simulink model "P2"  (R2019a)
settings: Solver=VariableStepAuto  StartTime=0.0  StopTime=50.0  RelTol=1e-3
libraries: simulink x8
settings Model: Creator=ADMIN  LastModifiedBy=ADMIN

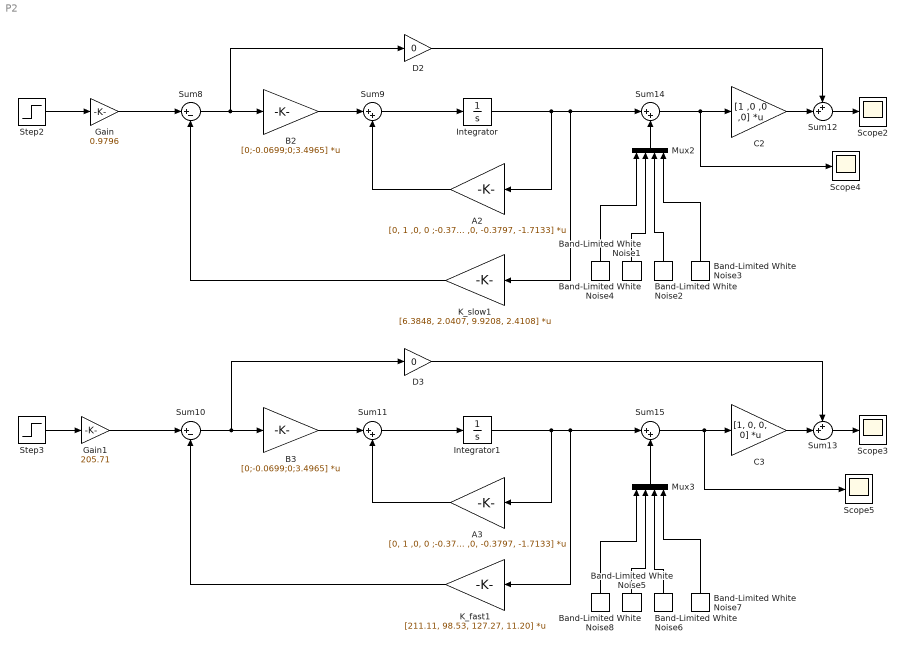
== system P2 ==
  A2 : Gain  Gain=[0, 1 ,0, 0 ;-0.378 ,0 ,7.0147 ,0.0343;0, 0, 0, 1; 18.9001 ,0, -0.3797, -1.7133]  Multiplication=Matrix(K*u) (u vector)
  A3 : Gain  Gain=[0, 1 ,0, 0 ;-0.378 ,0 ,7.0147 ,0.0343;0, 0, 0, 1; 18.9001 ,0, -0.3797, -1.7133]  Multiplication=Matrix(K*u) (u vector)
  B2 : Gain  Gain=[0;-0.0699;0;3.4965]  Multiplication=Matrix(K*u) (u vector)
  B3 : Gain  Gain=[0;-0.0699;0;3.4965]  Multiplication=Matrix(K*u) (u vector)
  Band-Limited White Noise1 : simulink/Sources/Band-Limited White Noise  Cov=[1e-5]  Ts=10  seed=2525
  Band-Limited White Noise2 : simulink/Sources/Band-Limited White Noise  Cov=[1e-5]  Ts=10  seed=[23341]
  Band-Limited White Noise3 : simulink/Sources/Band-Limited White Noise  Cov=[1e-5]  Ts=10  seed=[2342]
  Band-Limited White Noise4 : simulink/Sources/Band-Limited White Noise  Cov=[1e-5]  Ts=10  seed=[3]
  Band-Limited White Noise5 : simulink/Sources/Band-Limited White Noise  Cov=[1e-5]  Ts=10  seed=2525
  Band-Limited White Noise6 : simulink/Sources/Band-Limited White Noise  Cov=[1e-5]  Ts=10  seed=[23341]
  Band-Limited White Noise7 : simulink/Sources/Band-Limited White Noise  Cov=[1e-5]  Ts=10  seed=[2342]
  Band-Limited White Noise8 : simulink/Sources/Band-Limited White Noise  Cov=[1e-5]  Ts=10  seed=[3]
  C2 : Gain  Gain=[1 ,0 ,0 ,0]  Multiplication=Matrix(K*u) (u vector)
  C3 : Gain  Gain=[1, 0, 0, 0]  Multiplication=Matrix(K*u) (u vector)
  D2 : Gain  Gain=0
  D3 : Gain  Gain=0
  Gain : Gain  Gain=0.9796
  Gain1 : Gain  Gain=205.71
  Integrator : Integrator
  Integrator1 : Integrator
  K_fast1 : Gain  Gain=[211.11, 98.53, 127.27, 11.20]  Multiplication=Matrix(K*u) (u vector)
  K_slow1 : Gain  Gain=[6.3848, 2.0407, 9.9208, 2.4108]  Multiplication=Matrix(K*u) (u vector)
  Mux2 : Mux
  Mux3 : Mux
  Scope{2..5} (4 alike) : Scope
  Step2 : Step  Time=0  After=0.1  SampleTime=0
  Step3 : Step  Time=0  After=0.1  SampleTime=0
  Sum10 : Sum  Inputs=|+-
  Sum{9,11,14..15} (4 alike) : Sum  Inputs=|++
  Sum12 : Sum  Inputs=++|
  Sum13 : Sum  Inputs=++|
  Sum8 : Sum  Inputs=|+-
  wires:
  Sum8/1 -> B2/1, D2/1
  Sum11/1 -> Integrator1/1
  Gain/1 -> Sum8/1
  Step2/1 -> Gain/1
  Gain1/1 -> Sum10/1
  Step3/1 -> Gain1/1
  Sum13/1 -> Scope3/1
  C3/1 -> Sum13/2
  D2/1 -> Sum12/1
  C2/1 -> Sum12/2
  A2/1 -> Sum9/2
  Sum9/1 -> Integrator/1
  B2/1 -> Sum9/1
  K_slow1/1 -> Sum8/2
  A3/1 -> Sum11/2
  Sum12/1 -> Scope2/1
  B3/1 -> Sum11/1
  K_fast1/1 -> Sum10/2
  Sum10/1 -> B3/1, D3/1
  D3/1 -> Sum13/1
  Mux2/1 -> Sum14/2
  Band-Limited White Noise3/1 -> Mux2/4
  Band-Limited White Noise4/1 -> Mux2/1
  Sum14/1 -> Scope4/1, C2/1
  Band-Limited White Noise2/1 -> Mux2/3
  Integrator/1 -> A2/1, Sum14/1, K_slow1/1
  Integrator1/1 -> Sum15/1, K_fast1/1, A3/1
  Band-Limited White Noise6/1 -> Mux3/3
  Band-Limited White Noise5/1 -> Mux3/2
  Band-Limited White Noise8/1 -> Mux3/1
  Mux3/1 -> Sum15/2
  Sum15/1 -> Scope5/1, C3/1
  Band-Limited White Noise7/1 -> Mux3/4
  Band-Limited White Noise1/1 -> Mux2/2
